simulink library "ElectricPowerMotorCalculator"  (R2016b)
settings: Solver=VariableStepAuto  StartTime=0.0  StopTime=10.0  RelTol=1e-3
undefined symbols (not defined in the file or in its folder): backEMFConstant, motorResistance
libraries: ConversionsLibrary x1
settings Model: Creator=MARCH  LastModifiedBy=MARCH

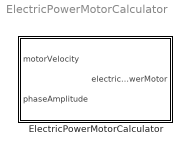
== system ElectricPowerMotorCalculator ==
  ElectricPowerMotorCalculator : Subsystem

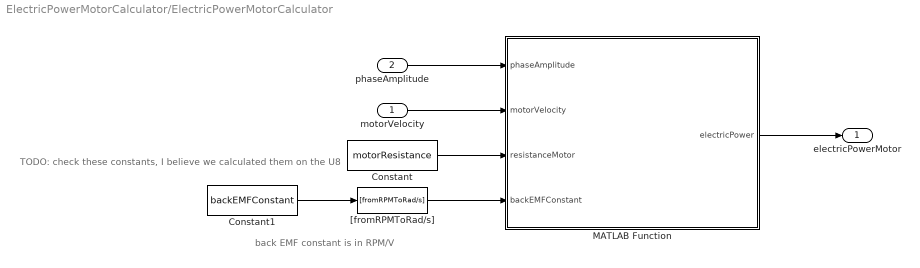
== system ElectricPowerMotorCalculator/ElectricPowerMotorCalculator ==
  note: TODO: check these constants, I believe we calculated them on the U8
  note: back EMF constant is in RPM/V
  motorVelocity : Inport
  phaseAmplitude : Inport  Port=2
  Constant : Constant  Value=motorResistance
  Constant1 : Constant  Value=backEMFConstant
  MATLAB Function : MATLAB Function  TreatAsAtomicUnit=on
  "[fromRPMToRad/s]" : ConversionsLibrary/[fromRPMToRad//s]
  electricPowerMotor : Outport
  wires:
  Constant/1 -> MATLAB Function/3(resistanceMotor)
  motorVelocity/1 -> MATLAB Function/2(motorVelocity)
  phaseAmplitude/1 -> MATLAB Function/1(phaseAmplitude)
  MATLAB Function/1(electricPower) -> electricPowerMotor/1
  Constant1/1 -> "[fromRPMToRad/s]"/1
  "[fromRPMToRad/s]"/1 -> MATLAB Function/4(backEMFConstant)

== matlab function ElectricPowerMotorCalculator/MATLAB Function ==
  data: phaseAmplitude input; electricPower output; motorVelocity input; resistanceMotor input; backEMFConstant input
function electricPower   = getElectricPowerMotor( phaseAmplitude, motorVelocity, resistanceMotor, backEMFConstant)
% wrapper for getElectricPowerMotor
electricPower = getElectricPowerMotor( phaseAmplitude, motorVelocity, resistanceMotor, backEMFConstant);
end
